simulink model "SingleTrack5statesV2"  (R2019b)
settings: Solver=FixedStepAuto  StartTime=0.0  StopTime=1000  FixedStep=Ts  MaxStep=Ts  MinStep=Ts/10  RelTol=1e-1
values from neighbouring files (symbols this model uses):
  car = Porsche928    [init.m]
  initBeta = 0    [init.m]
  initR = 0    [init.m]
  initV = 20    [init.m]
settings Model: Creator=efrem  LastModifiedBy=dominik
settings SolverCC: ZeroCrossAlgorithm=Adaptive
settings DataIOCC: ReturnWorkspaceOutputs=off
settings DebuggingCC: MaxConsecutiveZCsMsg=none  PregeneratedLibrarySubsystemCodeDiagnostic=none  ArithmeticOperatorsInVariantConditions=warning
settings SFSimCC: SimUseLocalCustomCode=off  CustomCodeUndefinedFunction=UseInterfaceOnly
settings RTWCC: RTWUseLocalCustomCode=off
settings CodeAppCC: StateflowObjectComments=on

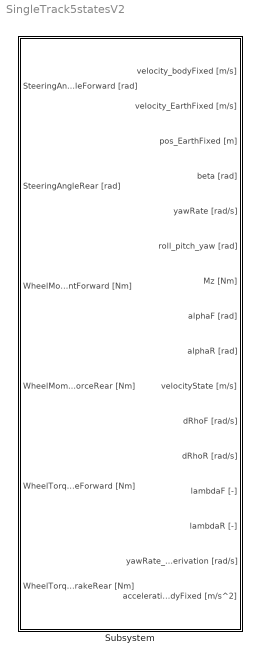
== system SingleTrack5statesV2 ==
  Subsystem : Subsystem

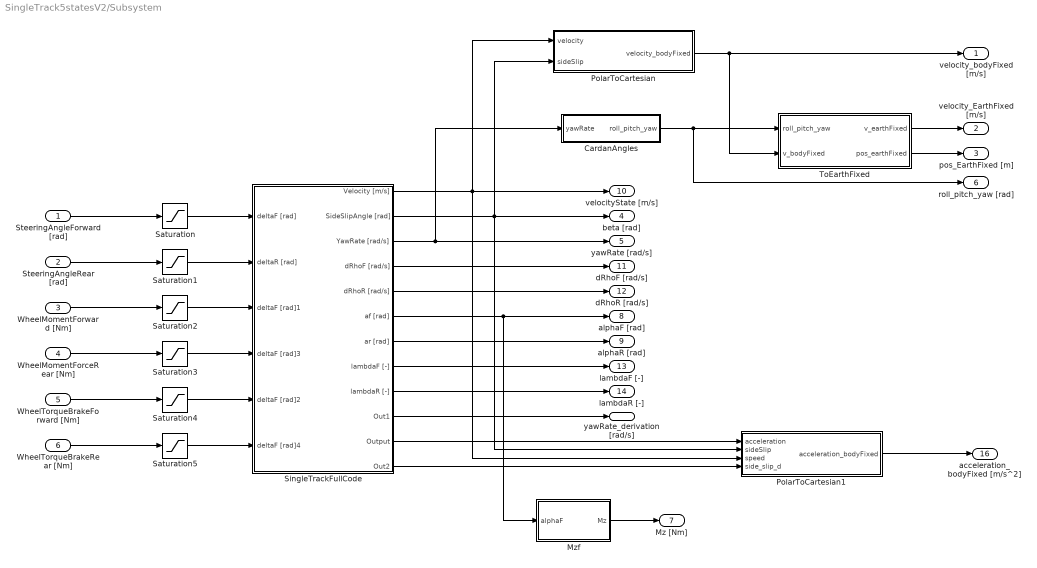
== system SingleTrack5statesV2/Subsystem ==
  SteeringAngleForward [rad] : Inport
  SteeringAngleRear [rad] : Inport  Port=2
  WheelMomentForward [Nm] : Inport  Port=3
  WheelMomentForceRear [Nm] : Inport  Port=4
  WheelTorqueBrakeForward [Nm] : Inport  Port=5
  WheelTorqueBrakeRear [Nm] : Inport  Port=6
  CardanAngles : Subsystem
  Mzf : Subsystem
  PolarToCartesian : Subsystem
  PolarToCartesian1 : Subsystem
  Saturation : Saturate  UpperLimit=pi/3  LowerLimit=-pi/3  ZeroCross=off
  Saturation1 : Saturate  UpperLimit=pi/3  LowerLimit=-pi/3  ZeroCross=off
  Saturation2 : Saturate  UpperLimit=2000  LowerLimit=0  ZeroCross=off
  Saturation3 : Saturate  UpperLimit=2000  LowerLimit=0  ZeroCross=off
  Saturation4 : Saturate  UpperLimit=5000  LowerLimit=0  ZeroCross=off
  Saturation5 : Saturate  UpperLimit=5000  LowerLimit=0  ZeroCross=off
  SingleTrackFullCode : Subsystem
  ToEarthFixed : Subsystem
  velocity_bodyFixed [m/s] : Outport  VectorParamsAs1DForOutWhenUnconnected=off
  velocity_EarthFixed [m/s] : Outport  Port=2  VectorParamsAs1DForOutWhenUnconnected=off
  pos_EarthFixed [m] : Outport  Port=3  VectorParamsAs1DForOutWhenUnconnected=off
  beta [rad] : Outport  Port=4  VectorParamsAs1DForOutWhenUnconnected=off
  yawRate [rad/s] : Outport  Port=5  VectorParamsAs1DForOutWhenUnconnected=off
  roll_pitch_yaw [rad] : Outport  Port=6  VectorParamsAs1DForOutWhenUnconnected=off
  Mz [Nm] : Outport  Port=7  VectorParamsAs1DForOutWhenUnconnected=off
  alphaF [rad] : Outport  Port=8  VectorParamsAs1DForOutWhenUnconnected=off
  alphaR [rad] : Outport  Port=9  VectorParamsAs1DForOutWhenUnconnected=off
  velocityState [m/s] : Outport  Port=10  VectorParamsAs1DForOutWhenUnconnected=off
  dRhoF [rad/s] : Outport  Port=11  VectorParamsAs1DForOutWhenUnconnected=off
  dRhoR [rad/s] : Outport  Port=12  VectorParamsAs1DForOutWhenUnconnected=off
  lambdaF [-] : Outport  Port=13  VectorParamsAs1DForOutWhenUnconnected=off
  lambdaR [-] : Outport  Port=14  VectorParamsAs1DForOutWhenUnconnected=off
  yawRate_derivation [rad/s] : Outport  Port=15  VectorParamsAs1DForOutWhenUnconnected=off
  acceleration_bodyFixed [m/s^2] : Outport  Port=16  VectorParamsAs1DForOutWhenUnconnected=off
  wires:
  SteeringAngleForward [rad]/1 -> Saturation/1
  WheelTorqueBrakeForward [Nm]/1 -> Saturation4/1
  SingleTrackFullCode/7(ar [rad]) -> alphaR [rad]/1
  SingleTrackFullCode/12(Out2) -> PolarToCartesian1/4(side_slip_d)
  ToEarthFixed/2(pos_earthFixed) -> pos_EarthFixed [m]/1
  CardanAngles/1(roll_pitch_yaw) -> ToEarthFixed/1(roll_pitch_yaw), roll_pitch_yaw [rad]/1
  WheelMomentForceRear [Nm]/1 -> Saturation3/1
  SingleTrackFullCode/9(lambdaR [-]) -> lambdaR [-]/1
  Mzf/1(Mz) -> Mz [Nm]/1
  SingleTrackFullCode/5(dRhoR [rad/s]) -> dRhoR [rad/s]/1
  Saturation3/1 -> SingleTrackFullCode/4(deltaF [rad]3)
  WheelTorqueBrakeRear [Nm]/1 -> Saturation5/1
  SingleTrackFullCode/6(af [rad]) -> alphaF [rad]/1, Mzf/1(alphaF)
  PolarToCartesian1/1(acceleration_bodyFixed) -> acceleration_bodyFixed [m/s^2]/1
  SingleTrackFullCode/4(dRhoF [rad/s]) -> dRhoF [rad/s]/1
  WheelMomentForward [Nm]/1 -> Saturation2/1
  SingleTrackFullCode/8(lambdaF [-]) -> lambdaF [-]/1
  SingleTrackFullCode/10(Out1) -> yawRate_derivation [rad/s]/1
  Saturation2/1 -> SingleTrackFullCode/3(deltaF [rad]1)
  Saturation5/1 -> SingleTrackFullCode/6(deltaF [rad]4)
  SingleTrackFullCode/2(SideSlipAngle [rad]) -> beta [rad]/1, PolarToCartesian1/2(sideSlip), PolarToCartesian/2(sideSlip)
  SingleTrackFullCode/11(Output) -> PolarToCartesian1/1(acceleration)
  SingleTrackFullCode/3(YawRate [rad/s]) -> yawRate [rad/s]/1, CardanAngles/1(yawRate)
  ToEarthFixed/1(v_earthFixed) -> velocity_EarthFixed [m/s]/1
  Saturation4/1 -> SingleTrackFullCode/5(deltaF [rad]2)
  SingleTrackFullCode/1(Velocity [m/s]) -> velocityState [m/s]/1, PolarToCartesian1/3(speed), PolarToCartesian/1(velocity)
  SteeringAngleRear [rad]/1 -> Saturation1/1
  PolarToCartesian/1(velocity_bodyFixed) -> velocity_bodyFixed [m/s]/1, ToEarthFixed/2(v_bodyFixed)
  Saturation1/1 -> SingleTrackFullCode/2(deltaR [rad])
  Saturation/1 -> SingleTrackFullCode/1(deltaF [rad])

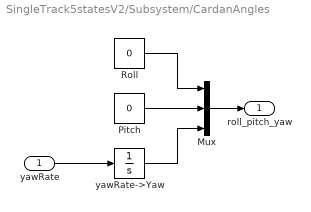
== system SingleTrack5statesV2/Subsystem/CardanAngles ==
  yawRate : Inport
  Mux : Mux  Inputs=3
  Pitch : Constant  Value=0
  Roll : Constant  Value=0
  yawRate->Yaw : Integrator
  roll_pitch_yaw : Outport  VectorParamsAs1DForOutWhenUnconnected=off
  wires:
  Pitch/1 -> Mux/2
  Roll/1 -> Mux/1
  Mux/1 -> roll_pitch_yaw/1
  yawRate->Yaw/1 -> Mux/3
  yawRate/1 -> yawRate->Yaw/1

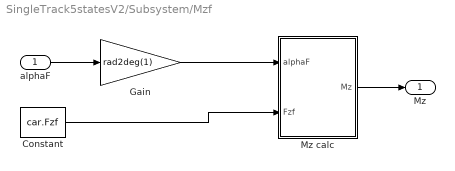
== system SingleTrack5statesV2/Subsystem/Mzf ==
  alphaF : Inport
  Constant : Constant  Value=car.Fzf
  Gain : Gain  Gain=rad2deg(1)
  Mz calc : MATLAB Function  TreatAsAtomicUnit=on
  Mz : Outport  VectorParamsAs1DForOutWhenUnconnected=off
  wires:
  Mz calc/1(Mz) -> Mz/1
  alphaF/1 -> Gain/1
  Constant/1 -> Mz calc/2(Fzf)
  Gain/1 -> Mz calc/1(alphaF)

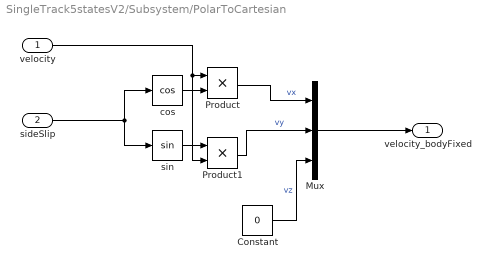
== system SingleTrack5statesV2/Subsystem/PolarToCartesian ==
  velocity : Inport
  sideSlip : Inport  Port=2
  Constant : Constant  Value=0
  Mux : Mux  Inputs=3
  Product : Product
  Product1 : Product
  cos : Trigonometry  Operator=cos
  sin : Trigonometry
  velocity_bodyFixed : Outport  VectorParamsAs1DForOutWhenUnconnected=off
  wires:
  Product/1 -> Mux/1  "vx"
  velocity/1 -> Product/1, Product1/2
  sin/1 -> Product1/1
  sideSlip/1 -> cos/1, sin/1
  Product1/1 -> Mux/2  "vy"
  cos/1 -> Product/2
  Constant/1 -> Mux/3  "vz"
  Mux/1 -> velocity_bodyFixed/1

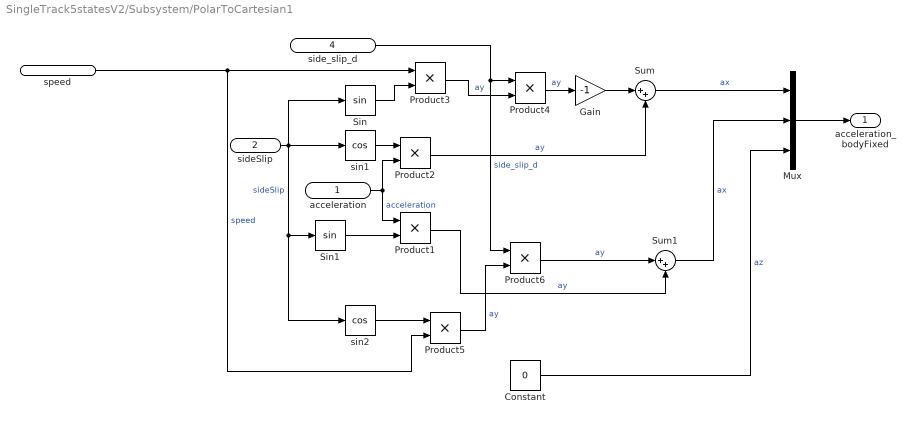
== system SingleTrack5statesV2/Subsystem/PolarToCartesian1 ==
  acceleration : Inport
  sideSlip : Inport  Port=2
  speed : Inport  Port=3
  side_slip_d : Inport  Port=4
  Constant : Constant  Value=0
  Gain : Gain  Gain=-1
  Mux : Mux  Inputs=3
  Product{1..6} (6 alike) : Product
  Sin : Trigonometry
  Sin1 : Trigonometry
  Sum : Sum  Inputs=|++
  Sum1 : Sum  Inputs=|++
  sin1 : Trigonometry  Operator=cos
  sin2 : Trigonometry  Operator=cos
  acceleration_bodyFixed : Outport  VectorParamsAs1DForOutWhenUnconnected=off
  wires:
  Product4/1 -> Gain/1  "ay"
  sin1/1 -> Product2/1
  Sin/1 -> Product3/2
  Product2/1 -> Sum/2  "ay"
  Gain/1 -> Sum/1
  Product3/1 -> Product4/2  "ay"
  Mux/1 -> acceleration_bodyFixed/1
  Constant/1 -> Mux/3  "az"
  Sum/1 -> Mux/1  "ax"
  Product5/1 -> Product6/2  "ay"
  side_slip_d/1 -> Product6/1, Product4/1  "side_slip_d"
  Product1/1 -> Sum1/2  "ay"
  acceleration/1 -> Product2/2, Product1/1  "acceleration"
  Product6/1 -> Sum1/1  "ay"
  sideSlip/1 -> sin1/1, sin2/1, Sin1/1, Sin/1  "sideSlip"
  speed/1 -> Product5/2, Product3/1  "speed"
  Sum1/1 -> Mux/2  "ax"
  Sin1/1 -> Product1/2
  sin2/1 -> Product5/1

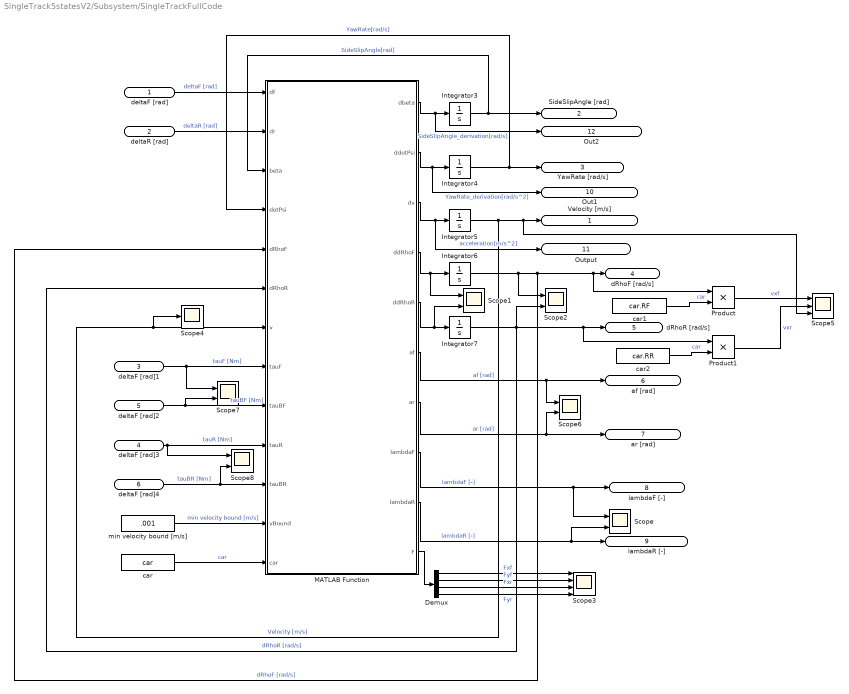
== system SingleTrack5statesV2/Subsystem/SingleTrackFullCode ==
  deltaF [rad] : Inport
  deltaR [rad] : Inport  Port=2
  deltaF [rad]1 : Inport  Port=3
  deltaF [rad]3 : Inport  Port=4
  deltaF [rad]2 : Inport  Port=5
  deltaF [rad]4 : Inport  Port=6
  Demux : Demux
  Integrator3 : Integrator  InitialCondition=initBeta  UpperSaturationLimit=pi/2  LowerSaturationLimit=-pi/2  ZeroCross=off
  Integrator4 : Integrator  InitialCondition=initR  UpperSaturationLimit=pi/2  LowerSaturationLimit=-pi/2  ZeroCross=off
  Integrator5 : Integrator  InitialCondition=initV  UpperSaturationLimit=pi/2  LowerSaturationLimit=-pi/2  ZeroCross=off
  Integrator6 : Integrator  InitialCondition=initV/car.RF  LowerSaturationLimit=0  ZeroCross=off
  Integrator7 : Integrator  InitialCondition=initV/car.RR  LowerSaturationLimit=0  ZeroCross=off
  MATLAB Function : MATLAB Function  TreatAsAtomicUnit=on
  Product : Product
  Product1 : Product
  Scope{,1..2,6..8} (6 alike) : Scope  NumInputPorts=2
  Scope3 : Scope  NumInputPorts=4
  Scope4 : Scope
  Scope5 : Scope  NumInputPorts=3
  car : Constant  Value=car  OutDataTypeStr=Bus: car_bus
  car1 : Constant  Value=car.RF  OutDataTypeStr=double
  car2 : Constant  Value=car.RR  OutDataTypeStr=double
  min velocity bound [m/s] : Constant  Value=.001
  Velocity [m/s] : Outport  VectorParamsAs1DForOutWhenUnconnected=off
  SideSlipAngle [rad] : Outport  Port=2  VectorParamsAs1DForOutWhenUnconnected=off
  YawRate [rad/s] : Outport  Port=3  VectorParamsAs1DForOutWhenUnconnected=off
  dRhoF [rad/s] : Outport  Port=4  VectorParamsAs1DForOutWhenUnconnected=off
  dRhoR [rad/s] : Outport  Port=5  VectorParamsAs1DForOutWhenUnconnected=off
  af [rad] : Outport  Port=6  VectorParamsAs1DForOutWhenUnconnected=off
  ar [rad] : Outport  Port=7  VectorParamsAs1DForOutWhenUnconnected=off
  lambdaF [-] : Outport  Port=8  VectorParamsAs1DForOutWhenUnconnected=off
  lambdaR [-] : Outport  Port=9  VectorParamsAs1DForOutWhenUnconnected=off
  Out1 : Outport  Port=10  VectorParamsAs1DForOutWhenUnconnected=off
  Output : Outport  Port=11  VectorParamsAs1DForOutWhenUnconnected=off
  Out2 : Outport  Port=12  VectorParamsAs1DForOutWhenUnconnected=off
  wires:
  deltaF [rad]/1 -> MATLAB Function/1(df)  "deltaF [rad]"
  deltaR [rad]/1 -> MATLAB Function/2(dr)  "deltaR [rad]"
  deltaF [rad]1/1 -> Scope7/1, MATLAB Function/8(tauF)  "tauF [Nm]"
  deltaF [rad]3/1 -> Scope8/1, MATLAB Function/10(tauR)  "tauR [Nm]"
  car/1 -> MATLAB Function/13(car)  "car"
  min velocity bound [m/s]/1 -> MATLAB Function/12(vBound)  "min velocity bound [m/s]"
  MATLAB Function/1(dbeta) -> Out2/1, Integrator3/1  "SideSlipAngle_derivation[rad/s]"
  Integrator3/1 -> SideSlipAngle [rad]/1, MATLAB Function/3(beta)  "SideSlipAngle[rad]"
  MATLAB Function/2(ddotPsi) -> Out1/1, Integrator4/1  "YawRate_derivation[rad/s^2]"
  Integrator4/1 -> YawRate [rad/s]/1, MATLAB Function/4(dotPsi)  "YawRate[rad/s]"
  Integrator5/1 -> Scope4/1, MATLAB Function/7(v), Scope5/3, Velocity [m/s]/1  "Velocity [m/s]"
  MATLAB Function/4(ddRhoF) -> Scope1/1, Integrator6/1
  MATLAB Function/5(ddRhoR) -> Scope1/2, Integrator7/1
  Integrator7/1 -> Scope2/2, Product1/1, dRhoR [rad/s]/1, MATLAB Function/6(dRhoR)  "dRhoR [rad/s]"
  deltaF [rad]2/1 -> Scope7/2, MATLAB Function/9(tauBF)  "tauBF [Nm]"
  deltaF [rad]4/1 -> Scope8/2, MATLAB Function/11(tauBR)  "tauBR [Nm]"
  MATLAB Function/6(af) -> Scope6/1, af [rad]/1  "af [rad]"
  MATLAB Function/7(ar) -> Scope6/2, ar [rad]/1  "ar [rad]"
  Integrator6/1 -> Scope2/1, Product/1, dRhoF [rad/s]/1, MATLAB Function/5(dRhoF)  "dRhoF [rad/s]"
  MATLAB Function/8(lambdaF) -> Scope/1, lambdaF [-]/1  "lambdaF [-]"
  MATLAB Function/9(lambdaR) -> Scope/2, lambdaR [-]/1  "lambdaR [-]"
  MATLAB Function/3(dv) -> Output/1, Integrator5/1  "acceleration[m/s^2]"
  MATLAB Function/10(F) -> Demux/1
  Demux/1 -> Scope3/1  "Fxf"
  Demux/2 -> Scope3/2  "Fyf"
  Demux/3 -> Scope3/3  "Fxr"
  Demux/4 -> Scope3/4  "Fyr"
  car1/1 -> Product/2  "car"
  car2/1 -> Product1/2  "car"
  Product/1 -> Scope5/1  "vxf"
  Product1/1 -> Scope5/2  "vxr"

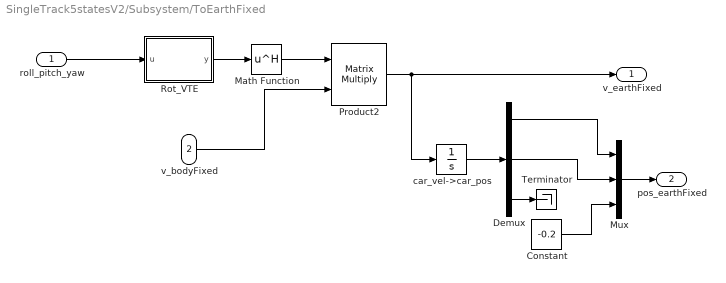
== system SingleTrack5statesV2/Subsystem/ToEarthFixed ==
  roll_pitch_yaw : Inport
  v_bodyFixed : Inport  Port=2
  Constant : Constant  Value=-0.2
  Demux : Demux  Outputs=3
  Math Function : Math  Operator=hermitian  SaturateOnIntegerOverflow=on
  Mux : Mux  Inputs=3
  Product2 : Product  Multiplication=Matrix(*)
  Rot_VTE : MATLAB Function  TreatAsAtomicUnit=on
  Terminator : Terminator
  car_vel->car_pos : Integrator
  v_earthFixed : Outport  VectorParamsAs1DForOutWhenUnconnected=off
  pos_earthFixed : Outport  Port=2  VectorParamsAs1DForOutWhenUnconnected=off
  wires:
  v_bodyFixed/1 -> Product2/2
  Product2/1 -> v_earthFixed/1, car_vel->car_pos/1
  Constant/1 -> Mux/3
  Mux/1 -> pos_earthFixed/1
  car_vel->car_pos/1 -> Demux/1
  Demux/2 -> Mux/2
  Demux/1 -> Mux/1
  Math Function/1 -> Product2/1
  roll_pitch_yaw/1 -> Rot_VTE/1(u)
  Rot_VTE/1(y) -> Math Function/1
  Demux/3 -> Terminator/1

== matlab function SingleTrack5statesV2/Subsystem/Mzf/Mz calc ==
  data: alphaF input; Mz output; Fzf input
function Mz = fcn(alphaF, Fzf)
Bz = .15;
Cz = 2.3;
Dz = -.05 * Fzf;
Ez = -10;
Mz = Dz*sin((Cz*atan(Bz*alphaF - Ez*(Bz*alphaF - atan(Bz*alphaF)))));

== matlab function SingleTrack5statesV2/Subsystem/SingleTrackFullCode/MATLAB Function ==
  data: df input; dbeta output; dr input; beta input; dotPsi input; dRhoF input; dRhoR input; v input; tauF input; tauBF input; tauR input; tauBR input; vBound input; car input; ddotPsi output; dv output; ddRhoF output; ddRhoR output; af output; ar output; lambdaF output; lambdaR output; F output
function [dbeta, ddotPsi, dv, ddRhoF, ddRhoR, af, ar, lambdaF, lambdaR,F]= SingleTrackFullModelFunctionCode(df, dr, beta, dotPsi, dRhoF, dRhoR, v, tauF, tauBF, tauR, tauBR, vBound, car)

    %% parse parameters 
    lf = car.LF;
    lr = car.LR;
    m = car.Mass;
    Fzf = car.Fzf;
    Fzr = car.Fzb;
    Jr = car.JR;
    Jf = car.JF;
    Rr = car.RR;
    Rf = car.RF;
    Iz = car.Iz;
    D = car.Pacejka.D;
    B = car.Pacejka.B;
    C = car.Pacejka.C;
    E = car.Pacejka.E;
    Dx = car.Pacejka.Dx;
    Bx = car.Pacejka.Bx;
    Cx = car.Pacejka.Cx;
    Ex = car.Pacejka.Ex;
    %% apply deadzone for the wheel velocity
    
    if (dRhoF<vBound*Rf && dRhoF >= 0) 
        dRhoF = dRhoF+vBound*Rf;
    elseif (dRhoR > -vBound*Rf && dRhoR <0)
        dRhoF = dRhoF - vBound*Rf;
    end
    
    if (dRhoR<vBound*Rr && dRhoR >= 0) 
        dRhoR = dRhoR+vBound*Rr;
    elseif (dRhoR > -vBound*Rr && dRhoR <0)
        dRhoR = dRhoR- vBound*Rr;
    end
    
    %% apply deadzone for the velocity
    if(v < vBound && v >= 0) 
		v = v+vBound;
	elseif (v > -vBound && v <0)
        v = v-vBound;
    end
    
    %% Long. velocities on the wheels
    vxf = v*cos(beta)*cos(df)+(v*sin(beta)+lf*dotPsi)*sin(df); %součet ryclostí na kolo v ose x a y
    vxr = v*cos(beta)*cos(dr)+(v*sin(beta)-lr*dotPsi)*sin(dr); %součet rychlostí na kolo v ose x a y
    
    %% Slip Ratios
    lambdaF = (dRhoF*Rf - vxf)/max(dRhoF*Rf,abs(vxf));
    lambdaR = (dRhoR*Rr - vxr)/max(dRhoR*Rr,abs(vxr));
    
    lambdaF(lambdaF>1) = 1;
    lambdaF(lambdaF<-1) = -1;
    lambdaR(lambdaR>1) = 1;
    lambdaR(lambdaR<-1) = -1;
    
    
    %% Slip angles
    af = -atan2((v*sin(beta)+lf*dotPsi)*cos(df)-v*cos(beta)*sin(df),...
        abs((v*sin(beta)+lf*dotPsi)*sin(df)+ v*cos(beta)*cos(df)));
    
    ar = -atan2((v*sin(beta)-lr*dotPsi)*cos(dr)-v*cos(beta)*sin(dr),...
        abs((v*sin(beta)-lr*dotPsi)*sin(dr)+ v*cos(beta)*cos(dr)));
    
    %% Pacejka Raw
    af_deg = rad2deg(af); % only in case of my parametrization for degrees
    ar_deg = rad2deg(ar);
    
    Fyf0 = D * Fzf * sin(C * atan(B*af_deg - E*(B*af_deg - atan(B*af_deg))));
    Fyr0 = D * Fzr * sin(C * atan(B*ar_deg - E*(B*ar_deg - atan(B*ar_deg))));

    Fxf0 = Dx * Fzf * sin(Cx * atan(Bx*lambdaF - Ex*(Bx*lambdaF - atan(Bx*lambdaF))));
    Fxr0 = Dx * Fzr * sin(Cx * atan(Bx*lambdaR - Ex*(Bx*lambdaR - atan(Bx*lambdaR))));
    
    %% Traction Ellipse Forward
    
    betaStar = acos(abs(lambdaF)/sqrt(lambdaF^2 + sin(af)^2));

    % friction coefficients
    mu_x_act = Fxf0/Fzf;
    mu_y_act = Fyf0/Fzf;

    mu_x_max = Dx;
    mu_y_max = D;

    mu_x =         1/sqrt((1/mu_x_act)^2 + (tan(betaStar)/mu_y_max)^2 );
    mu_y = tan(betaStar)/sqrt((1/mu_x_max)^2 + (tan(betaStar)/mu_y_act)^2 );

    Fxf = abs(mu_x/mu_x_act)*Fxf0;
    Fyf = abs(mu_y/mu_y_act)*Fyf0;

    if isnan(Fxf)
        Fxf = 0;
    end

    if isnan(Fyf)
        Fyf = 0;
    end

    if Fzf == 0
        Fxf = Fxf0;
        Fyf = Fyf0;
    end
    
    %% Traction Ellipse Rear
    betaStar = acos(abs(lambdaR)/sqrt(lambdaR^2 + sin(ar)^2));
    % friction coefficients
    mu_x_act = Fxr0/Fzr;
    mu_y_act = Fyr0/Fzr;

    mu_x_max = Dx;
    mu_y_max = D;

    mu_x =         1/sqrt((1/mu_x_act)^2 + (tan(betaStar)/mu_y_max)^2 );
    mu_y = tan(betaStar)/sqrt((1/mu_x_max)^2 + (tan(betaStar)/mu_y_act)^2 );

    Fxr = abs(mu_x/mu_x_act)*Fxr0;
    Fyr = abs(mu_y/mu_y_act)*Fyr0;


    if isnan(Fxr)
        Fxr = 0;
    end

    if isnan(Fyr)
        Fyr = 0;
    end

    if Fzr == 0
        Fxr = Fxr0;
        Fyr = Fyr0;
    end
    
    %% Steering angles projection and Dynamics
    
    SAP = [cos(df), -sin(df), cos(dr), -sin(dr);...
        sin(df), cos(df), sin(dr), cos(dr);...
        lf*sin(df), lf*cos(df), -lr*sin(dr), -lr*cos(dr)];

    F = [Fxf; Fyf; Fxr; Fyr];

    RotDyn = [-sin(beta), cos(beta), 0;...
        cos(beta), sin(beta), 0;...
        0, 0, 1];
    
    Dyn = RotDyn * (SAP * F);
    
    % parse to motions
    lat = Dyn(1);
    long = Dyn(2);
    rot = Dyn(3);
    
	%% Body states
    dbeta = - dotPsi + lat/m/v;
    dv = (long/m) - 0.001*v^2; % upravit
    ddotPsi = rot/Iz; 
	
	%% Wheel models
    %{
    Vof = sqrt(9.81*Rf); Vor = sqrt(9.81*Rr); % i have no idea why... i guess it can change gain?
    Vrf = Rf*dRhoF; Vrr = Rr*dRhoR;% Rf  a Rr by měl být nahrazen efektivní hodnotou Rfe a Rre.
    lf = (0.001+ 0.001*abs(vxf/Vof)+ 0.0001*(vxf/Vof)^4);%random as fuck i coud not find correct parameters
    lr = (0.001+ 0.001*abs(vxr/Vof)+ 0.0001*(vxr/Vof)^4);%random as fuck i coud not find correct parameters
    Frf = Fzf*lf; 
    Frr = Fzr*lr;
    Myf = Fxf*(Rf-Rf) + Frf*Rf*atan2(Vrf,Vof); % Rf by měl být nahrazen efektivní hodnotou Rfe..pro zatim nahrazeno konstantou
    Myr = Fxr*(Rr-Rr) + Frr*Rr*atan2(Vrr,Vor); % Rf by měl být nahrazen efektivní hodnotou Rfe..pro zatim nahrazeno konstantou
    ddRhoF = (tauF - Rf*Fxf - sign(dRhoF)*tauBF -Myf)/Jf;
    ddRhoR = (tauR - Rr*Fxr - sign(dRhoR)*tauBR -Myr)/Jr;
    %}
     ddRhoR = (tauR - Rr*Fxr - sign(dRhoR)*tauBR -Dx*(dRhoR*Rr-vxr)/Rr)/Jr;
     ddRhoF = (tauF - Rf*Fxf - sign(dRhoF)*tauBF -Dx*(dRhoF*Rf-vxf)/Rf)/Jf;
%     ddRhoR = (tauR - Rr*Fxr - sign(dRhoR)*tauBR -Dx*(dRhoR*Rr-vxr)/Rr)/Jr;
%     ddRhoF = (tauF -Rf*Fxf - sign(dRhoF)*tauBF)/Jf;
%     ddRhoR = (tauR - Rr*Fxr - sign(dRhoR)*tauBR)/Jr;
end

== matlab function SingleTrack5statesV2/Subsystem/ToEarthFixed/Rot_VTE ==
  data: u input; y output
function y = fcn(u)
y = Rot_VTE(u);
